simulink model "Learn_EngineStartStop_11252014"  (R2014b)
settings: Solver=ode23  StartTime=0.0  StopTime=100  MaxStep=0.1  RelTol=1e-3
libraries: fl_lib x8, nesl_utility x5, sdl_lib x1
settings Model: PauseTimes=31.6  Creator=RaymondSutjiono  LastModifiedBy=RaymondSutjiono

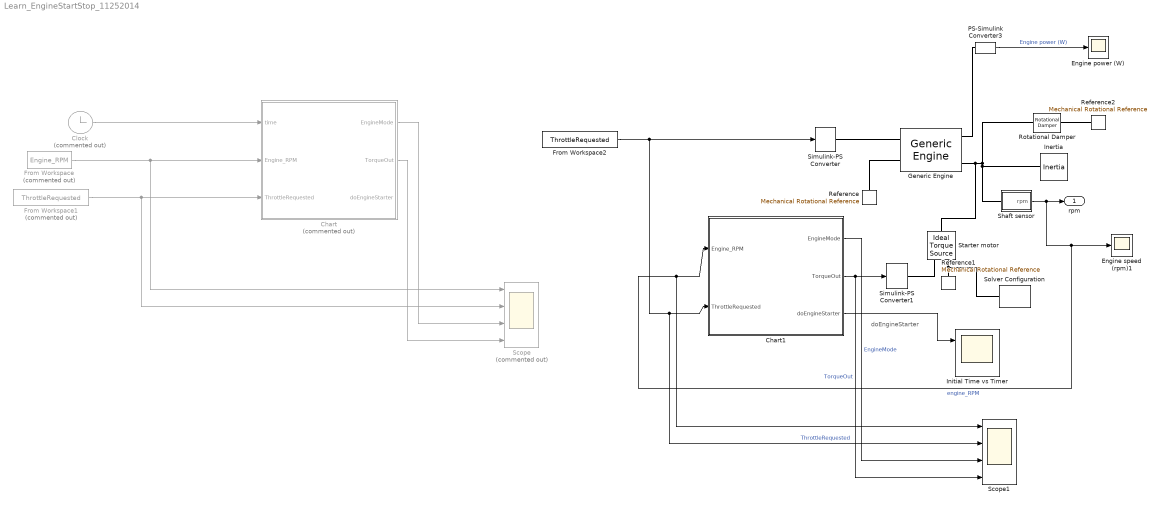
== system Learn_EngineStartStop_11252014 ==
  note: doEngineStarter
  Chart : Stateflow chart  Commented=on  TreatAsAtomicUnit=on
  Chart1 : Stateflow chart  TreatAsAtomicUnit=on
  Clock : Clock  Commented=on
  Engine power (W) : Scope
      settings: TimeRange=150  YMin=-50000  YMax=150000  MaxDataPoints=500000  SampleTime=0.1
  Engine speed (rpm)1 : Scope
      settings: TimeRange=150  YMin=0  YMax=4000  SaveName=ScopeData6  MaxDataPoints=500000  SampleTime=0.1
  From Workspace : FromWorkspace  Commented=on  VariableName=Engine_RPM  SampleTime=0
  From Workspace1 : FromWorkspace  Commented=on  VariableName=ThrottleRequested  SampleTime=0
  From Workspace2 : FromWorkspace  VariableName=ThrottleRequested  SampleTime=0
  Generic Engine : sdl_lib/Engines/Generic Engine  model_parameterization=1  engine_type=1  P_max=10 HP  w_P_max=8000 rpm  w_max=9000 rpm  w_min=500 rpm  w_tab=[ 500 1000 2e+3 3e+3 4e+3 5e+3 6e+3 7e+3 ] rpm  trq_tab=[ 380 380 380 380 350 280 200 80 ] N*m  pwr_tab=[ 2e+4 4e+4 7.8e+4 1.2e+5 1.45e+5 1.48e+5 1.25e+5 6e+4 ] W  interp_method=1  model_inertia=0  inertia=0.08 kg*m^2  initial_velocity=800 rpm  model_time_constant=1  time_constant=0.4 s  T0=0  w_thr=100 rpm  idle_speed=0  idle_speed_reference=1000 rpm  tau_controller=1 s  idle_w_thr=1 rpm  fc_model=1  fc_per_rev=25 mg/rev  displaced_volume=400 cm^3  rev_per_cycle=2  fc_w_tab=[ 1000 2e+3 3e+3 4e+3 5e+3 6e+3 ] rpm  fc_trq_tab=[ 0 80 160 200 240 320 360 400 ] N*m  fc_tab=[ 0.5 0.9 1.4 1.6 1.9 2.7 3.4 4.4; 1 1.7 2.7 3.1 3.6 5 6 7.4; 1.4 2.7 4 4.8 5.6 7.5 8.5 10.5; 2 3.6 5.8 6.7 8 10.4 11.7 13.3; 2.5 4.8 7.9 9.4 10.8 14 16.2 18.6; 3.1 6 10.3 11.9 13.8 18.4 22 26.5 ] g/s  bmep_tab=[ 0 250 500 625 750 1000 1.15e+3 1.25e+3 ] kPa  bsfc_tab=[ 410 380 300 280 270 290 320 380; 410 370 290 270 260 270 285 320; 415 380 290 275 265 270 270 300; 420 390 310 290 285 280 280 285; 430 410 340 320 310 300 310 320; 450 430 370 340 330 330 350 380 ] g/hr/kW  fc_interp_method=1
  Inertia : fl_lib/Mechanical/Rotational Elements/Inertia  inertia=0.1 kg*m^2  w_specify=off  w_priority=High  w=0 rad/s  t_specify=off  t_priority=High  t=0 N*m
  Initial Time vs Timer : Scope  NumInputPorts=2
      settings: TimeRange=100  YMin=0~-1  YMax=1~1  SaveName=ScopeData3  MaxDataPoints=500000  SampleTime=0.1
  PS-Simulink Converter3 : nesl_utility/PS-Simulink Converter  PhysicalDomain=network_engine_domain  SubClassName=ps_output  LeftPortType=input  RightPortType=output  PseudoPeriodic=off  Frequencies=[]  Unit=W  AffineConversion=off
  Reference : fl_lib/Mechanical/Rotational Elements/Mechanical Rotational Reference
  Reference1 : fl_lib/Mechanical/Rotational Elements/Mechanical Rotational Reference
  Reference2 : fl_lib/Mechanical/Rotational Elements/Mechanical Rotational Reference
  Rotational Damper : fl_lib/Mechanical/Rotational Elements/Rotational Damper  D=0.02 N*m/(rad/s)  w_specify=off  w_priority=High  w=0 rad/s  t_specify=off  t_priority=High  t=0 N*m
  Scope : Scope  Commented=on  NumInputPorts=4
      settings: YMin=0~0~1~0  YMax=10000~1~3~5
  Scope1 : Scope  NumInputPorts=4
      settings: YMin=0~0~1~0  YMax=5000~1~3~10  SaveName=ScopeData2
  Shaft sensor : Subsystem
  Simulink-PS Converter1 : nesl_utility/Simulink-PS Converter  PhysicalDomain=network_engine_domain  SubClassName=ps_input  LeftPortType=input  RightPortType=output  PseudoPeriodic=off  Frequencies=[]  NoiseDistribution=none  NoiseParameters=[]  Unit=N*m  AffineConversion=off  InputFiltering=on  SimscapeFilterOrder=1  InputFilterTimeConstant=0.001  UdotUserProvided=1
  Simulink-PS Converter : nesl_utility/Simulink-PS Converter  PhysicalDomain=network_engine_domain  SubClassName=ps_input  LeftPortType=input  RightPortType=output  PseudoPeriodic=off  Frequencies=[]  NoiseDistribution=none  NoiseParameters=[]  Unit=1  AffineConversion=off  InputFiltering=off  SimscapeFilterOrder=1  InputFilterTimeConstant=.001  UdotUserProvided=[]
  Solver Configuration : nesl_utility/Solver Configuration  PhysicalDomain=network_engine_domain  SubClassName=solver  LeftPortType=input  RightPortType=generic  Accelerate=off  Tones=[]  Harmonics=[]  SimulateNoise=off  Profile=off  UseLocalSampling=off  EnableSwitchedLinearOptims=on  FrequencyDomain=off  UseCCode=off  RelTol=0.001  AbsTol=1e-06  MinStep=1e-09  ToWorkspace=off  DoDC=off  ResidualTolerance=1e-09  UseLocalSolver=on  LocalSolverChoice=NE_BACKWARD_EULER_ADVANCER  LocalSolverSampleTime=0.001  DoFixedCost=on  MaxNonlinIter=3  MaxModeIter=2  LinearAlgebra=Sparse  DelaysMemoryBudget=1024  AutomaticFiltering=on  FilteringTimeConstant=0.001
  Starter motor : fl_lib/Mechanical/Mechanical Sources/Ideal Torque Source
  rpm : Outport
  wires:
  Clock/1 -> Chart/1(time)
  From Workspace1/1 -> Chart/3(ThrottleRequested), Scope/2
  From Workspace/1 -> Scope/1, Chart/2(Engine_RPM)
  Chart/1(EngineMode) -> Scope/3
  Chart/2(TorqueOut) -> Scope/4
  PS-Simulink Converter3/1 -> Engine power (W)/1  "Engine power (W)"
  Shaft sensor/1(rpm) -> Scope1/1, Chart1/1(Engine_RPM), Engine speed (rpm)1/1, rpm/1  "engine_RPM"
  Chart1/2(TorqueOut) -> Scope1/4, Simulink-PS Converter1/1  "TorqueOut"
  From Workspace2/1 -> Scope1/2, Chart1/2(ThrottleRequested), Simulink-PS Converter/1  "ThrottleRequested"
  Chart1/1(EngineMode) -> Scope1/3  "EngineMode"
  Chart1/3(doEngineStarter) -> Initial Time vs Timer/1
  connections:
  Starter motor/LConn1 -- Generic Engine/RConn3 -- Shaft sensor/LConn1 -- Inertia/LConn1 -- Rotational Damper/LConn1
  Starter motor/RConn2 -- Solver Configuration/RConn1 -- Reference1/LConn1
  Simulink-PS Converter1/RConn1 -- Starter motor/RConn1
  Generic Engine/RConn1 -- PS-Simulink Converter3/LConn1
  Reference/LConn1 -- Generic Engine/LConn2
  Simulink-PS Converter/RConn1 -- Generic Engine/LConn1
  Rotational Damper/RConn1 -- Reference2/LConn1

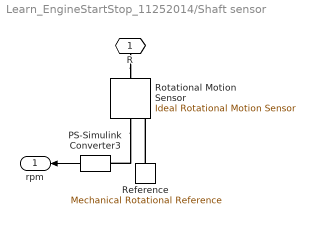
== system Learn_EngineStartStop_11252014/Shaft sensor ==
  PS-Simulink Converter3 : nesl_utility/PS-Simulink Converter  PhysicalDomain=network_engine_domain  SubClassName=ps_output  LeftPortType=input  RightPortType=output  PseudoPeriodic=off  Frequencies=[]  Unit=rpm  AffineConversion=off
  Reference : fl_lib/Mechanical/Rotational Elements/Mechanical Rotational Reference
  Rotational Motion Sensor : fl_lib/Mechanical/Mechanical Sensors/Ideal Rotational Motion Sensor  offset=0 rad
  R : PMIOPort  Port=1  Side=Left
  rpm : Outport
  wires:
  PS-Simulink Converter3/1 -> rpm/1
  connections:
  Rotational Motion Sensor/RConn2 -- PS-Simulink Converter3/LConn1
  Reference/LConn1 -- Rotational Motion Sensor/RConn1
  R/RConn1 -- Rotational Motion Sensor/LConn1

== stateflow chart Learn_EngineStartStop_11252014/Chart ==
  state ENGINE_STOP
    entry:
    EngineMode  = STOP;
  state ENGINE_StartRequest
    entry:
    EngineMode = StartRequest;
    IntialTimer = time;
    during:
    if(time - IntialTimer < 1)
    doEngineStarter = 1;
    end
    if doEngineStarter
    TorqueOut = 5;
    else
    TorqueOut = 0;
    end
  state ENGINE_Run
    entry:
    EngineMode = Run;
    doEngineStarter = 0;
    TorqueOut = 0;
  (default) -> ENGINE_STOP
  ENGINE_Run -> ENGINE_STOP : [ThrottleRequested< 0.1 && ...
      | Engine_RPM < 800]
  ENGINE_STOP -> ENGINE_StartRequest : [Engine_RPM < 800 && ...
      | ThrottleRequested > 0.1]
  ENGINE_StartRequest -> ENGINE_Run : [Engine_RPM > 800]
  data: time input double; EngineMode output; TorqueOut output; Engine_RPM input; ThrottleRequested input; IntialTimer local; doEngineStarter output; StartRequest constant double =2; Run constant double =3; STOP constant double =1

== stateflow chart Learn_EngineStartStop_11252014/Chart1 ==
  state ENGINE_STOP
    entry:
    EngineMode  = STOP;
  state ENGINE_StartRequest
    entry:
    EngineMode = StartRequest;
    during:
    if before(1,sec)
    doEngineStarter = 1;
    else
    doEngineStarter = 0;
    end
    if doEngineStarter
    TorqueOut = 10;
    else
    TorqueOut = 0;
    end
  state ENGINE_Run
    entry:
    EngineMode = Run;
    doEngineStarter = 0;
    TorqueOut = 0;
  (default) -> ENGINE_STOP
  ENGINE_Run -> ENGINE_STOP : [ThrottleRequested< 0.1 && ...
      | Engine_RPM < 800]
  ENGINE_StartRequest -> ENGINE_STOP [order 2] : [Engine_RPM <800 && ...
      | doEngineStarter ==0 &&...
      | after(5,sec)]
  ENGINE_StartRequest -> ENGINE_STOP [commented out] : [Engine_RPM <800 && ...
      | doEngineStarter ==0 &&...
      | TimeDiff > 5]
  ENGINE_STOP -> ENGINE_StartRequest : [Engine_RPM < 800 && ...
      | ThrottleRequested > 0.1 &&...
      | after(2,sec)]
  ENGINE_StartRequest -> ENGINE_Run [order 1] : [Engine_RPM > 800]
  data: EngineMode output; TorqueOut output; Engine_RPM input; ThrottleRequested input; doEngineStarter output; StartRequest constant double =2; Run constant double =3; STOP constant double =1
